simulink library "cdsRms"  (Simulink 6.2)
settings Model: LastModifiedBy=rolf

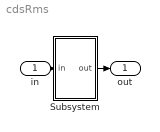
== system cdsRms ==
  in : Inport  Port=1  LatchInput=off
  Subsystem : Subsystem
  out : Outport
  wires:
  Subsystem/1(out) -> out/1
  in/1 -> Subsystem/1(in)

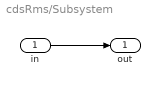
== system cdsRms/Subsystem ==
  in : Inport  Port=1  LatchInput=off
  out : Outport
  wires:
  in/1 -> out/1
